simulink model "em_field_check"  (R2025a)
settings: Solver=FixedStepDiscrete  StartTime=0.0  StopTime=3.0  FixedStep=P.dt  RelTol=1e-3
InitFcn:
  | em_ensure_init;
libraries: simulink x1
settings Model: Creator=Li  LastModifiedBy=Li

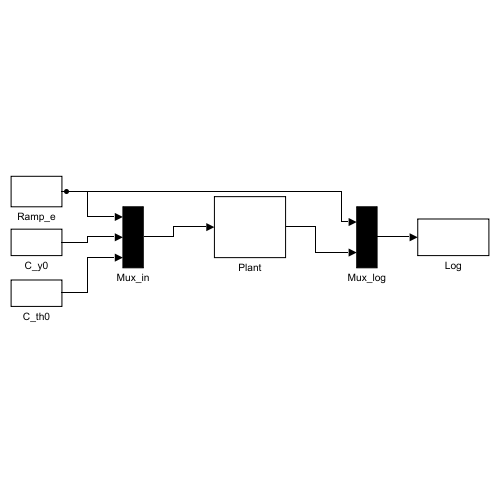
[thumbnail: Simulink's stored preview of the top-level diagram]
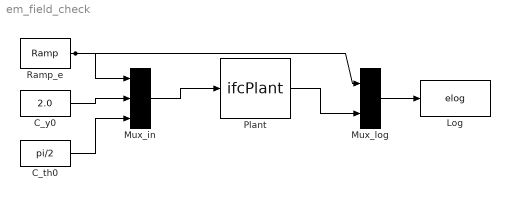
== system em_field_check ==
  C_th0 : Constant  Value=pi/2
  C_y0 : Constant  Value=2.0
  Log : ToWorkspace  VariableName=elog  SaveFormat=Structure With Time  SampleTime=-1
  Mux_in : Mux  Inputs=3
  Mux_log : Mux  Inputs=2
  Plant : MATLABFcn  MATLABFcn=ifcPlant  OutputDimensions=4
  Ramp_e : simulink/Sources/Ramp  slope=0.1  start=0  InitialOutput=-0.15
  wires:
  Ramp_e/1 -> Mux_in/1, Mux_log/1
  C_y0/1 -> Mux_in/2
  C_th0/1 -> Mux_in/3
  Mux_in/1 -> Plant/1
  Plant/1 -> Mux_log/2
  Mux_log/1 -> Log/1
